simulink model "QPSK"  (Simulink 7.2)
settings: Solver=ode45  StartTime=0.0  StopTime=20  RelTol=1e-3
StopFcn:
  | QPSK_RX_StopFcn
libraries: simulink_extras x3, dsparch4 x2, commrandsrc2 x1
settings Model: Creator=usuario  LastModifiedBy=USUARIO
settings OptimizationCC: InitFltsAndDblsToZero=on
settings DebuggingCC: SaveWithParameterizedLinksMsg=none  SignalResolutionControl=TryResolveAllWithWarning  MultiTaskDSMMsg=warning  MultiTaskCondExecSysMsg=none
settings RTWCC: IncludeERTFirstTime=on
settings GRTTargetCC: TargetFcnLib=ansi_tfl_tmw.mat

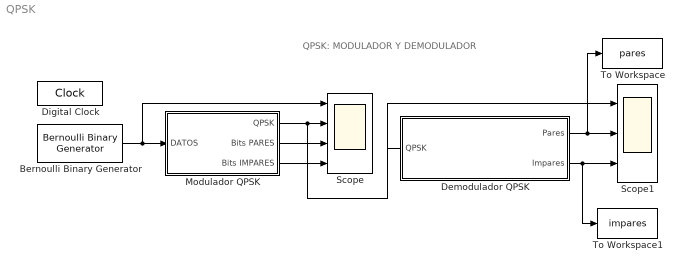
== system QPSK ==
  note: QPSK: MODULADOR Y DEMODULADOR
  Bernoulli Binary Generator : commrandsrc2/Bernoulli Binary Generator  DialogController=commDDGCreate  DialogControllerArgs=DataTag0  SystemSampleTime=-1  P=0.5  seed=61  Ts=.5  frameBased=off  sampPerFrame=1  orient=off  outDataType=double
  Demodulador QPSK : Subsystem
  Digital Clock : DigitalClock  SampleTime=0.001
  Modulador QPSK : Subsystem
  Scope : Scope  NumInputPorts=4
      settings: YMin=-5~-5~-5~-3  YMax=5~5~5~3  SampleInput=on
  Scope1 : Scope  NumInputPorts=3
      settings: YMin=-5~-5~-5  YMax=5~5~5  SaveName=ScopeData2  SampleInput=on
  To Workspace : ToWorkspace  VariableName=pares  SampleTime=1/100  SaveFormat=Array
  To Workspace1 : ToWorkspace  VariableName=impares  SampleTime=1/100  SaveFormat=Array
  wires:
  Modulador QPSK/1(QPSK) -> Scope/2, Demodulador QPSK/1(QPSK), Scope1/1
  Bernoulli Binary Generator/1 -> Modulador QPSK/1(DATOS), Scope/1
  Modulador QPSK/2(Bits PARES) -> Scope/3
  Modulador QPSK/3(Bits IMPARES) -> Scope/4
  Demodulador QPSK/2(Impares) -> Scope1/3, To Workspace1/1
  Demodulador QPSK/1(Pares) -> Scope1/2, To Workspace/1

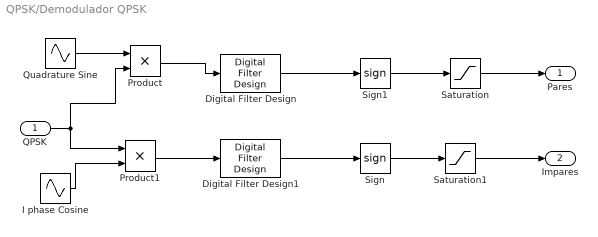
== system QPSK/Demodulador QPSK ==
  QPSK : Inport  OutDataType=sfix(16)  OutScaling=2^0
  Digital Filter Design : dsparch4/Digital Filter Design  SystemSampleTime=-1  mwdsp_browser_bugfix_var=off
  Digital Filter Design1 : dsparch4/Digital Filter Design  SystemSampleTime=-1  mwdsp_browser_bugfix_var=off
  I phase Cosine : Sin  Frequency=2*pi*4  Phase=pi  Samples=100  SampleTime=1/100  Offset=25
  Product : Product  OutDataType=sfix(16)  OutScaling=2^0  SampleTime=1/200  RndMeth=Zero
  Product1 : Product  OutDataType=sfix(16)  OutScaling=2^0  SampleTime=1/200  RndMeth=Zero
  Quadrature Sine : Sin  Frequency=2*pi*4  Phase=pi/2  Samples=100  SampleTime=1/100  Offset=50
  Saturation : Saturate  UpperLimit=1  LowerLimit=0
  Saturation1 : Saturate  UpperLimit=1  LowerLimit=0
  Sign : Signum
  Sign1 : Signum
  Pares : Outport  OutDataType=sfix(16)  OutScaling=2^0
  Impares : Outport  Port=2  OutDataType=sfix(16)  OutScaling=2^0
  wires:
  Quadrature Sine/1 -> Product/1
  QPSK/1 -> Product1/1, Product/2
  I phase Cosine/1 -> Product1/2
  Product1/1 -> Digital Filter Design1/1
  Product/1 -> Digital Filter Design/1
  Digital Filter Design/1 -> Sign1/1
  Digital Filter Design1/1 -> Sign/1
  Sign1/1 -> Saturation/1
  Saturation/1 -> Pares/1
  Sign/1 -> Saturation1/1
  Saturation1/1 -> Impares/1

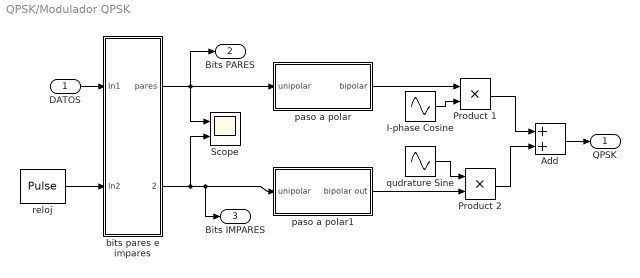
== system QPSK/Modulador QPSK ==
  DATOS : Inport  OutDataType=sfix(16)  OutScaling=2^0
  Add : Sum  OutDataType=sfix(16)  OutScaling=2^-10
  "I-phase Cosine " : Sin  Frequency=2*pi*4  Phase=pi/2  SampleTime=0.01
  Product 1 : Product  OutDataType=sfix(16)  OutScaling=2^0  RndMeth=Zero
  Product 2 : Product  OutDataType=sfix(16)  OutScaling=2^0  RndMeth=Zero
  Scope : Scope  NumInputPorts=2
      settings: YMin=-5~-5  YMax=5~5  SampleInput=on
  bits pares e impares : Subsystem
  paso a polar : Subsystem
  paso a polar1 : Subsystem
  qudrature Sine : Sin  Frequency=2*pi*4  Phase=pi  SampleTime=0.01
  reloj : DiscretePulseGenerator  PulseType=Time based  Period=1  PulseWidth=50
  QPSK : Outport  OutDataType=sfix(16)  OutScaling=2^0
  Bits PARES : Outport  Port=2  OutDataType=sfix(16)  OutScaling=2^0
  Bits IMPARES : Outport  Port=3  OutDataType=sfix(16)  OutScaling=2^0
  wires:
  Add/1 -> QPSK/1
  DATOS/1 -> bits pares e impares/1(In1)
  bits pares e impares/2(impares) -> Scope/2, paso a polar1/1(unipolar), Bits IMPARES/1
  reloj/1 -> bits pares e impares/2(In2)
  "I-phase Cosine "/1 -> Product 1/2
  qudrature Sine/1 -> Product 2/1
  paso a polar/1(bipolar) -> Product 1/1
  paso a polar1/1(bipolar out) -> Product 2/2
  Product 1/1 -> Add/1
  Product 2/1 -> Add/2
  bits pares e impares/1(pares) -> paso a polar/1(unipolar), Scope/1, Bits PARES/1

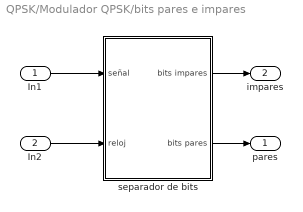
== system QPSK/Modulador QPSK/bits pares e impares ==
  In1 : Inport  OutDataType=sfix(16)  OutScaling=2^0
  In2 : Inport  Port=2  OutDataType=sfix(16)  OutScaling=2^0
  separador de bits : Subsystem
  pares : Outport  OutDataType=sfix(16)  OutScaling=2^0
  impares : Outport  Port=2  OutDataType=sfix(16)  OutScaling=2^0
  wires:
  In2/1 -> separador de bits/2(reloj)
  In1/1 -> separador de bits/1(señal)
  separador de bits/1(bits impares) -> impares/1
  separador de bits/2(bits pares) -> pares/1

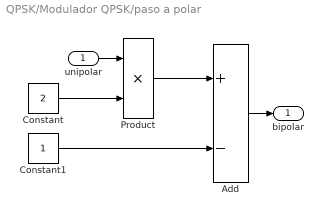
== system QPSK/Modulador QPSK/paso a polar ==
  unipolar : Inport  OutDataType=sfix(16)  OutScaling=2^0
  Add : Sum  Inputs=+-  OutDataType=sfix(16)  OutScaling=2^-10
  Constant : Constant  Value=2  OutDataType=sfix(16)  OutScaling=2^0
  Constant1 : Constant  OutDataType=sfix(16)  OutScaling=2^0
  Product : Product  OutDataType=sfix(16)  OutScaling=2^0  RndMeth=Zero
  bipolar : Outport  OutDataType=sfix(16)  OutScaling=2^0
  wires:
  Add/1 -> bipolar/1
  unipolar/1 -> Product/1
  Constant1/1 -> Add/2
  Product/1 -> Add/1
  Constant/1 -> Product/2

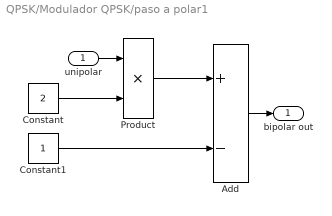
== system QPSK/Modulador QPSK/paso a polar1 ==
  unipolar : Inport  OutDataType=sfix(16)  OutScaling=2^0
  Add : Sum  Inputs=+-  OutDataType=sfix(16)  OutScaling=2^-10
  Constant : Constant  Value=2  OutDataType=sfix(16)  OutScaling=2^0
  Constant1 : Constant  OutDataType=sfix(16)  OutScaling=2^0
  Product : Product  OutDataType=sfix(16)  OutScaling=2^0  RndMeth=Zero
  bipolar out : Outport  OutDataType=sfix(16)  OutScaling=2^0
  wires:
  Constant/1 -> Product/2
  Product/1 -> Add/1
  Constant1/1 -> Add/2
  unipolar/1 -> Product/1
  Add/1 -> bipolar out/1

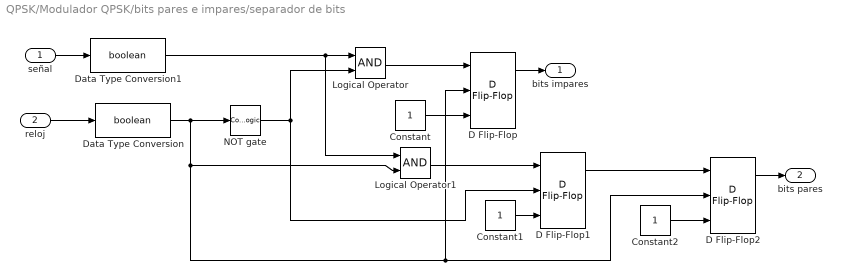
== system QPSK/Modulador QPSK/bits pares e impares/separador de bits ==
  señal : Inport  OutDataType=sfix(16)  OutScaling=2^0
  reloj : Inport  Port=2  OutDataType=sfix(16)  OutScaling=2^0
  Constant : Constant  OutDataTypeMode=boolean  OutDataType=sfix(16)  OutScaling=2^0  OutDataTypeStr=boolean
  Constant1 : Constant  OutDataTypeMode=boolean  OutDataType=sfix(16)  OutScaling=2^0  OutDataTypeStr=boolean
  Constant2 : Constant  OutDataTypeMode=boolean  OutDataType=sfix(16)  OutScaling=2^0  OutDataTypeStr=boolean
  D Flip-Flop : simulink_extras/Flip Flops/D Flip-Flop  SystemSampleTime=-1
  D Flip-Flop1 : simulink_extras/Flip Flops/D Flip-Flop  SystemSampleTime=-1
  D Flip-Flop2 : simulink_extras/Flip Flops/D Flip-Flop  SystemSampleTime=-1
  Data Type Conversion : DataTypeConversion  OutDataTypeMode=boolean  OutDataType=sfix(16)  OutScaling=2^0  OutDataTypeStr=boolean
  Data Type Conversion1 : DataTypeConversion  OutDataTypeMode=boolean  OutDataType=sfix(16)  OutScaling=2^0  OutDataTypeStr=boolean
  Logical Operator : Logic  AllPortsSameDT=off  OutDataTypeMode=boolean  OutDataTypeStr=boolean
  Logical Operator1 : Logic  AllPortsSameDT=off  OutDataTypeMode=boolean  OutDataTypeStr=boolean
  NOT gate : CombinatorialLogic  TruthTable=[1;0]
  bits impares : Outport  OutDataType=sfix(16)  OutScaling=2^0
  bits pares : Outport  Port=2  OutDataType=sfix(16)  OutScaling=2^0
  wires:
  D Flip-Flop1/1 -> D Flip-Flop2/1
  D Flip-Flop2/1 -> bits pares/1
  Constant2/1 -> D Flip-Flop2/3
  Constant/1 -> D Flip-Flop/3
  Constant1/1 -> D Flip-Flop1/3
  D Flip-Flop/1 -> bits impares/1
  Data Type Conversion/1 -> D Flip-Flop/2, D Flip-Flop2/2, Logical Operator1/2, NOT gate/1
  Logical Operator1/1 -> D Flip-Flop1/1
  Logical Operator/1 -> D Flip-Flop/1
  Data Type Conversion1/1 -> Logical Operator1/1, Logical Operator/1
  NOT gate/1 -> D Flip-Flop1/2, Logical Operator/2
  reloj/1 -> Data Type Conversion/1
  señal/1 -> Data Type Conversion1/1
